simulink model "mech_fceng_vr"  (Simulink 7.1)
settings: Solver=ode45  StartTime=0.0  StopTime=inf  RelTol=1e-3  AbsTol=1e-4
PreLoadFcn:
  | mech_fceng_init;load mech_fceng_images;
InitFcn:
  | mech_slider_open(gcs);
values from neighbouring files (symbols this model uses):
  AirRo = 1.2E-3    (= 0.0012)    [mech_sceng_init.m]
  Cv = 3    [mech_sceng_init.m]
  G = 9.81    [mech_motorcycle_data.m]    (also in mech_sceng_init.m = 1.4)
  Pa = 1033.34    [mech_sceng_init.m]
  Q = 46816    [mech_sceng_init.m]
  R = y([30:p],2)./y([30:p],1)    [mech_car_handling_sweep.m]    (also in mech_flexible_beamelement.m = [1  0  0; mech_sceng_init.m = 5; mech_toroid_setup.m = 10)
  Ta = 25    [mech_sceng_init.m]
  Vo = pi*R*R*14    (= 1099.55742876)    [mech_sceng_init.m]
  Vtdc = pi*R*R*2    (= 157.079632679)    [mech_sceng_init.m]
libraries: mblibv1 x47, simulink x3, simulink_extras x1
(part 2 of 2)

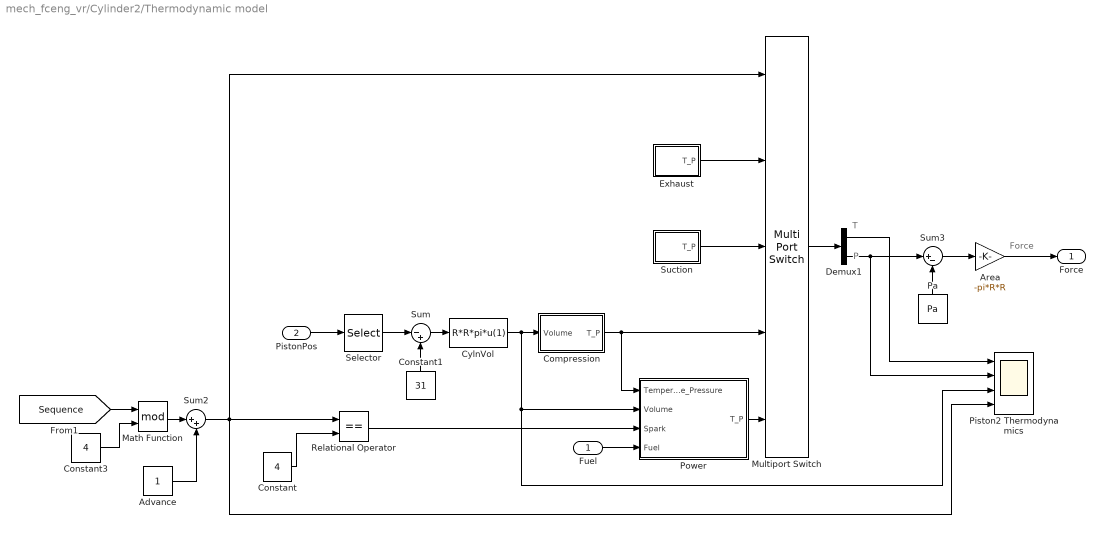
== system mech_fceng_vr/Cylinder2/Thermodynamic model ==
  note: Force
  note: P
  note: T
  Fuel : Inport  OutDataType=sfix(16)  OutScaling=2^0
  PistonPos : Inport  Port=2  OutDataType=sfix(16)  OutScaling=2^0
  Advance : Constant  OutDataType=sfix(16)  OutScaling=2^0
  Area : Gain  Gain=-pi*R*R  ParameterDataType=sfix(16)  ParameterScaling=2^0  OutDataType=sfix(16)  OutScaling=2^0  SaturateOnIntegerOverflow=on  OutDataTypeStr=Inherit: Same as input  ParamDataTypeStr=Inherit: Same as input
  Compression : Subsystem
  Constant : Constant  Value=4  OutDataType=sfix(16)  OutScaling=2^0
  Constant1 : Constant  Orientation=up  Value=31  OutDataType=sfix(16)  OutScaling=2^0
  Constant3 : Constant  Value=4  OutDataType=sfix(16)  OutScaling=2^0
  CylnVol : Fcn  Expr=R*R*pi*u(1)
  Demux1 : Demux  Outputs=2
  Exhaust : Subsystem  TreatAsAtomicUnit=on
  Math Function : Math  Operator=mod  OutDataType=sfix(16)  OutScaling=2^0  SaturateOnIntegerOverflow=on
  Multiport Switch : MultiPortSwitch  Inputs=4  InputSameDT=on
  Pa : Constant  Orientation=up  Value=Pa  OutDataType=sfix(16)  OutScaling=2^0
  Piston2 Thermodynamics : Scope  NumInputPorts=4
      settings: YMin=20~0~0~1  YMax=160~90000~1100~4
  Power : Subsystem
  Relational Operator : RelationalOperator  Operator===  ZeroCross=off  InputSameDT=on
  Selector : Selector  InputPortWidth=3  IndexOptions=Index vector (dialog)  Indices=2  OutputSizes=1
  Suction : Subsystem  TreatAsAtomicUnit=on
  Sum : Sum  Inputs=|-+  OutDataType=sfix(16)  OutScaling=2^0  SaturateOnIntegerOverflow=on  InputSameDT=on  OutDataTypeStr=Inherit: Same as first input
  Sum2 : Sum  Inputs=|++  OutDataType=sfix(16)  OutScaling=2^0  SaturateOnIntegerOverflow=on  InputSameDT=on  OutDataTypeStr=Inherit: Same as first input
  Sum3 : Sum  Inputs=|+-  OutDataType=sfix(16)  OutScaling=2^0  SaturateOnIntegerOverflow=on  InputSameDT=on  OutDataTypeStr=Inherit: Same as first input
  Force : Outport  OutDataType=sfix(16)  OutScaling=2^0
  wires:
  Sum2/1 -> Piston2 Thermodynamics/4, Multiport Switch/1, Relational Operator/1
  [Sequence] -> Math Function/1
  Advance/1 -> Sum2/2
  Math Function/1 -> Sum2/1
  Constant3/1 -> Math Function/2
  PistonPos/1 -> Selector/1
  Selector/1 -> Sum/1
  Relational Operator/1 -> Power/3(Spark)
  Area/1 -> Force/1
  Sum/1 -> CylnVol/1
  Constant/1 -> Relational Operator/2
  Demux1/1 -> Piston2 Thermodynamics/1
  Compression/1(T_P) -> Multiport Switch/4, Power/1(Temperature_Pressure)
  CylnVol/1 -> Piston2 Thermodynamics/3, Power/2(Volume), Compression/1(Volume)
  Constant1/1 -> Sum/2
  Fuel/1 -> Power/4(Fuel)
  Power/1(T_P) -> Multiport Switch/5
  Demux1/2 -> Piston2 Thermodynamics/2, Sum3/1
  Sum3/1 -> Area/1
  Pa/1 -> Sum3/2
  Multiport Switch/1 -> Demux1/1
  Exhaust/1(T_P) -> Multiport Switch/2
  Suction/1(T_P) -> Multiport Switch/3

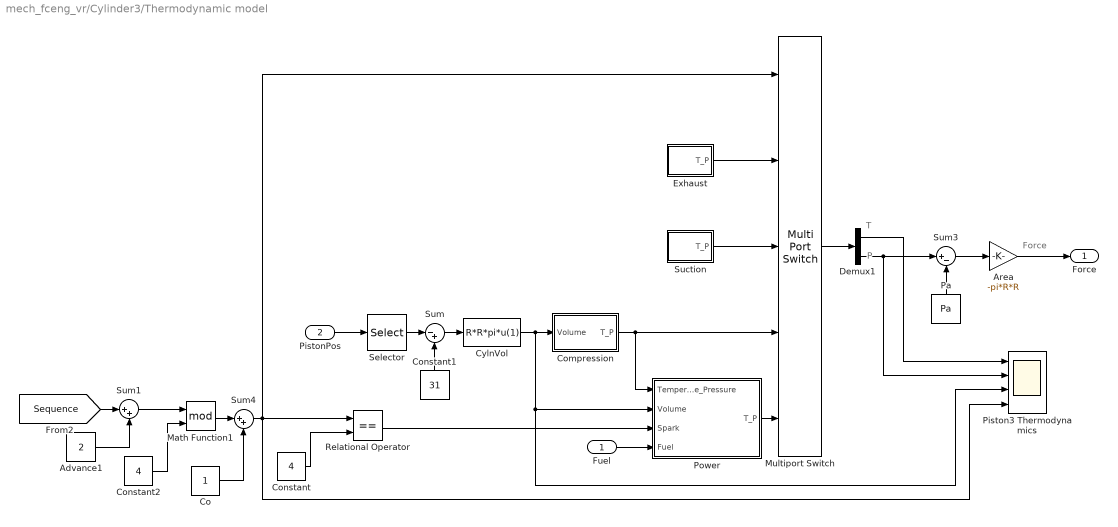
== system mech_fceng_vr/Cylinder3/Thermodynamic model ==
  note: Force
  note: P
  note: T
  Fuel : Inport  OutDataType=sfix(16)  OutScaling=2^0
  PistonPos : Inport  Port=2  OutDataType=sfix(16)  OutScaling=2^0
  Advance1 : Constant  Value=2  OutDataType=sfix(16)  OutScaling=2^0
  Area : Gain  Gain=-pi*R*R  ParameterDataType=sfix(16)  ParameterScaling=2^0  OutDataType=sfix(16)  OutScaling=2^0  SaturateOnIntegerOverflow=on  OutDataTypeStr=Inherit: Same as input  ParamDataTypeStr=Inherit: Same as input
  Co : Constant  OutDataType=sfix(16)  OutScaling=2^0
  Compression : Subsystem
  Constant : Constant  Value=4  OutDataType=sfix(16)  OutScaling=2^0
  Constant1 : Constant  Orientation=up  Value=31  OutDataType=sfix(16)  OutScaling=2^0
  Constant2 : Constant  Value=4  OutDataType=sfix(16)  OutScaling=2^0
  CylnVol : Fcn  Expr=R*R*pi*u(1)
  Demux1 : Demux  Outputs=2
  Exhaust : Subsystem  TreatAsAtomicUnit=on
  Math Function1 : Math  Operator=mod  OutDataType=sfix(16)  OutScaling=2^0  SaturateOnIntegerOverflow=on
  Multiport Switch : MultiPortSwitch  Inputs=4  InputSameDT=on
  Pa : Constant  Orientation=up  Value=Pa  OutDataType=sfix(16)  OutScaling=2^0
  Piston3 Thermodynamics : Scope  NumInputPorts=4
      settings: TimeRange=20  YMin=25~0~0~1  YMax=350~200000~1100~4
  Power : Subsystem
  Relational Operator : RelationalOperator  Operator===  ZeroCross=off  InputSameDT=on
  Selector : Selector  InputPortWidth=3  IndexOptions=Index vector (dialog)  Indices=2  OutputSizes=1
  Suction : Subsystem  TreatAsAtomicUnit=on
  Sum : Sum  Inputs=|-+  OutDataType=sfix(16)  OutScaling=2^0  SaturateOnIntegerOverflow=on  InputSameDT=on  OutDataTypeStr=Inherit: Same as first input
  Sum1 : Sum  Inputs=|++  OutDataType=sfix(16)  OutScaling=2^0  SaturateOnIntegerOverflow=on  InputSameDT=on  OutDataTypeStr=Inherit: Same as first input
  Sum3 : Sum  Inputs=|+-  OutDataType=sfix(16)  OutScaling=2^0  SaturateOnIntegerOverflow=on  InputSameDT=on  OutDataTypeStr=Inherit: Same as first input
  Sum4 : Sum  Inputs=|++  OutDataType=sfix(16)  OutScaling=2^0  SaturateOnIntegerOverflow=on  InputSameDT=on  OutDataTypeStr=Inherit: Same as first input
  Force : Outport  OutDataType=sfix(16)  OutScaling=2^0
  wires:
  Advance1/1 -> Sum1/2
  [Sequence] -> Sum1/1
  Sum1/1 -> Math Function1/1
  Co/1 -> Sum4/2
  Math Function1/1 -> Sum4/1
  Constant2/1 -> Math Function1/2
  Sum4/1 -> Piston3 Thermodynamics/4, Multiport Switch/1, Relational Operator/1
  PistonPos/1 -> Selector/1
  Selector/1 -> Sum/1
  Relational Operator/1 -> Power/3(Spark)
  Area/1 -> Force/1
  Sum/1 -> CylnVol/1
  Constant/1 -> Relational Operator/2
  Demux1/1 -> Piston3 Thermodynamics/1
  Compression/1(T_P) -> Multiport Switch/4, Power/1(Temperature_Pressure)
  CylnVol/1 -> Piston3 Thermodynamics/3, Power/2(Volume), Compression/1(Volume)
  Constant1/1 -> Sum/2
  Fuel/1 -> Power/4(Fuel)
  Power/1(T_P) -> Multiport Switch/5
  Demux1/2 -> Piston3 Thermodynamics/2, Sum3/1
  Sum3/1 -> Area/1
  Pa/1 -> Sum3/2
  Multiport Switch/1 -> Demux1/1
  Exhaust/1(T_P) -> Multiport Switch/2
  Suction/1(T_P) -> Multiport Switch/3

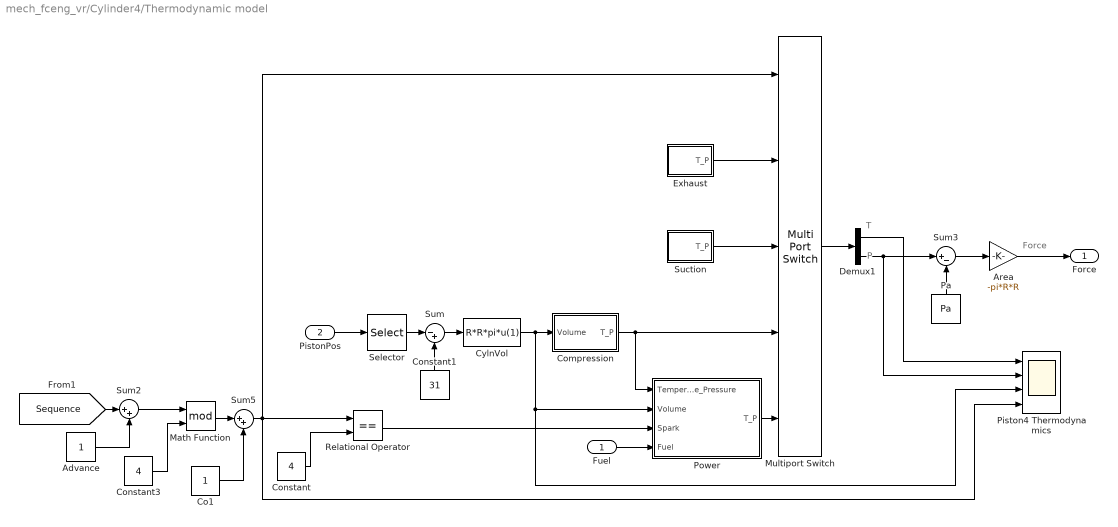
== system mech_fceng_vr/Cylinder4/Thermodynamic model ==
  note: T
  note: P
  note: Force
  Fuel : Inport  OutDataType=sfix(16)  OutScaling=2^0
  PistonPos : Inport  Port=2  OutDataType=sfix(16)  OutScaling=2^0
  Advance : Constant  OutDataType=sfix(16)  OutScaling=2^0
  Area : Gain  Gain=-pi*R*R  ParameterDataType=sfix(16)  ParameterScaling=2^0  OutDataType=sfix(16)  OutScaling=2^0  SaturateOnIntegerOverflow=on  OutDataTypeStr=Inherit: Same as input  ParamDataTypeStr=Inherit: Same as input
  Co1 : Constant  OutDataType=sfix(16)  OutScaling=2^0
  Compression : Subsystem
  Constant : Constant  Value=4  OutDataType=sfix(16)  OutScaling=2^0
  Constant1 : Constant  Orientation=up  Value=31  OutDataType=sfix(16)  OutScaling=2^0
  Constant3 : Constant  Value=4  OutDataType=sfix(16)  OutScaling=2^0
  CylnVol : Fcn  Expr=R*R*pi*u(1)
  Demux1 : Demux  Outputs=2
  Exhaust : Subsystem  TreatAsAtomicUnit=on
  Math Function : Math  Operator=mod  OutDataType=sfix(16)  OutScaling=2^0  SaturateOnIntegerOverflow=on
  Multiport Switch : MultiPortSwitch  Inputs=4  InputSameDT=on
  Pa : Constant  Orientation=up  Value=Pa  OutDataType=sfix(16)  OutScaling=2^0
  Piston4 Thermodynamics : Scope  NumInputPorts=4
      settings: YMin=0~0~0~1  YMax=4500~2.5e+006~1100~4
  Power : Subsystem
  Relational Operator : RelationalOperator  Operator===  ZeroCross=off  InputSameDT=on
  Selector : Selector  InputPortWidth=3  IndexOptions=Index vector (dialog)  Indices=2  OutputSizes=1
  Suction : Subsystem  TreatAsAtomicUnit=on
  Sum : Sum  Inputs=|-+  OutDataType=sfix(16)  OutScaling=2^0  SaturateOnIntegerOverflow=on  InputSameDT=on  OutDataTypeStr=Inherit: Same as first input
  Sum2 : Sum  Inputs=|++  OutDataType=sfix(16)  OutScaling=2^0  SaturateOnIntegerOverflow=on  InputSameDT=on  OutDataTypeStr=Inherit: Same as first input
  Sum3 : Sum  Inputs=|+-  OutDataType=sfix(16)  OutScaling=2^0  SaturateOnIntegerOverflow=on  InputSameDT=on  OutDataTypeStr=Inherit: Same as first input
  Sum5 : Sum  Inputs=|++  OutDataType=sfix(16)  OutScaling=2^0  SaturateOnIntegerOverflow=on  InputSameDT=on  OutDataTypeStr=Inherit: Same as first input
  Force : Outport  OutDataType=sfix(16)  OutScaling=2^0
  wires:
  Advance/1 -> Sum2/2
  [Sequence] -> Sum2/1
  Sum2/1 -> Math Function/1
  Co1/1 -> Sum5/2
  Math Function/1 -> Sum5/1
  Constant3/1 -> Math Function/2
  Suction/1(T_P) -> Multiport Switch/3
  Exhaust/1(T_P) -> Multiport Switch/2
  Multiport Switch/1 -> Demux1/1
  Pa/1 -> Sum3/2
  Sum3/1 -> Area/1
  Demux1/2 -> Sum3/1, Piston4 Thermodynamics/2
  Power/1(T_P) -> Multiport Switch/5
  Fuel/1 -> Power/4(Fuel)
  Constant1/1 -> Sum/2
  CylnVol/1 -> Compression/1(Volume), Power/2(Volume), Piston4 Thermodynamics/3
  Compression/1(T_P) -> Power/1(Temperature_Pressure), Multiport Switch/4
  Demux1/1 -> Piston4 Thermodynamics/1
  Constant/1 -> Relational Operator/2
  Sum/1 -> CylnVol/1
  Area/1 -> Force/1
  Relational Operator/1 -> Power/3(Spark)
  Selector/1 -> Sum/1
  PistonPos/1 -> Selector/1
  Sum5/1 -> Piston4 Thermodynamics/4, Relational Operator/1, Multiport Switch/1

== system mech_fceng_vr/Engine Block/Engine Timer ==
  Angle : Inport  Orientation=left  OutDataType=sfix(16)  OutScaling=2^0
  Constant : Constant  Orientation=left  Value=pi/4  OutDataType=sfix(16)  OutScaling=2^0
  Hit  Crossing2 : HitCross  Orientation=left  ZeroCross=off
  Ignition Control : Stateflow chart  Orientation=left  TreatAsAtomicUnit=on
  Sum : Sum  Orientation=left  Inputs=++|  OutDataType=sfix(16)  OutScaling=2^0  SaturateOnIntegerOverflow=on  InputSameDT=on  OutDataTypeStr=Inherit: Same as first input
  Trigonometric Function : Trigonometry  Orientation=left  Operator=cos
  tag scope: Sequence=global
  wires:
  Ignition Control/1(Sequence) -> [Sequence]
  Hit  Crossing2/1 -> Ignition Control/Trigger
  Trigonometric Function/1 -> Hit  Crossing2/1
  Sum/1 -> Ignition Control/1(CrankAngle), Trigonometric Function/1
  Constant/1 -> Sum/1
  Angle/1 -> Sum/2

== system mech_fceng_vr/Engine Block/Friction ==
  Angle : Inport  Orientation=left  OutDataType=sfix(16)  OutScaling=2^0
  Rate : Inport  Orientation=left  Port=2  OutDataType=sfix(16)  OutScaling=2^0
  Fcn : Fcn  Orientation=left  Expr=u < 0
  Gain : Gain  Orientation=left  Gain=1000  ParameterDataType=sfix(16)  ParameterScaling=2^0  OutDataType=sfix(16)  OutScaling=2^0  SaturateOnIntegerOverflow=on  OutDataTypeStr=Inherit: Same as input  ParamDataTypeStr=Inherit: Same as input
  Gain1 : Gain  Orientation=left  Gain=-200  ParameterDataType=sfix(16)  ParameterScaling=2^0  OutDataType=sfix(16)  OutScaling=2^0  SaturateOnIntegerOverflow=on  OutDataTypeStr=Inherit: Same as input  ParamDataTypeStr=Inherit: Same as input
  S-R Flip-Flop : simulink_extras/Flip Flops/S-R Flip-Flop  Orientation=left  SystemSampleTime=-1  initial_condition=0
  Sum1 : Sum  Orientation=left  Inputs=++|  OutDataType=sfix(16)  OutScaling=2^0  SaturateOnIntegerOverflow=on  InputSameDT=on  OutDataTypeStr=Inherit: Same as first input
  Torque : Outport  Orientation=left  OutDataType=sfix(16)  OutScaling=2^0
  tag scope: CrankSR=global
  wires:
  Sum1/1 -> Torque/1
  Angle/1 -> [CrankSR], Fcn/1
  Rate/1 -> Gain1/1
  Gain1/1 -> Sum1/1
  Gain/1 -> Sum1/2
  S-R Flip-Flop/2 -> Gain/1
  Fcn/1 -> S-R Flip-Flop/1

== system mech_fceng_vr/Cylinder1/Thermodynamic model/Compression ==
  note: Compression
  note: P
  note: T
  Volume : Inport  OutDataType=sfix(16)  OutScaling=2^0
  Mux : Mux  Inputs=2
  P : Fcn  Expr=Pa*(Vo/u(1))^G
  T : Fcn  Expr=Ta*(Vo/u(1))^(G-1)
  T_P : Outport  OutDataType=sfix(16)  OutScaling=2^0
  wires:
  Volume/1 -> P/1, T/1
  Mux/1 -> T_P/1
  P/1 -> Mux/2
  T/1 -> Mux/1

== system mech_fceng_vr/Cylinder1/Thermodynamic model/Exhaust ==
  note: Exhaust
  Mux : Mux  Inputs=2
  Pa : Constant  Value=Pa  OutDataType=sfix(16)  OutScaling=2^0
  Ta : Constant  Value=Ta  OutDataType=sfix(16)  OutScaling=2^0
  T_P : Outport  OutDataType=sfix(16)  OutScaling=2^0
  wires:
  Mux/1 -> T_P/1
  Ta/1 -> Mux/1
  Pa/1 -> Mux/2

== system mech_fceng_vr/Cylinder1/Thermodynamic model/Power ==
  Temperature_Pressure : Inport  OutDataType=sfix(16)  OutScaling=2^0
  Volume : Inport  Port=2  OutDataType=sfix(16)  OutScaling=2^0
  Spark : Inport  Port=3  OutDataType=sfix(16)  OutScaling=2^0
  Fuel : Inport  Port=4  OutDataType=sfix(16)  OutScaling=2^0
  Combustion : Subsystem  TreatAsAtomicUnit=on
  Demux1 : Demux  Outputs=2
  IC : InitialCondition  Value=[Ta;Pa]
  IdealExpansion : Subsystem  TreatAsAtomicUnit=on
  Mux : Mux  Inputs=2
  T_P : Outport  OutDataType=sfix(16)  OutScaling=2^0
  wires:
  Combustion/3(VolumeAfterCombustion) -> IdealExpansion/3(VolumeAfterCombustion)
  Combustion/1(TemperatureAfterCombustion) -> IdealExpansion/1(TemperatureAfterCombustion)
  IC/1 -> Demux1/1
  IdealExpansion/2(FPressure) -> Mux/2
  IdealExpansion/1(FTemperature) -> Mux/1
  Volume/1 -> Combustion/4(VolumeBeforeCombustion), IdealExpansion/4(IVolume)
  Combustion/2(PressureAfterCombustion) -> IdealExpansion/2(PressureAfterCombustion)
  Demux1/2 -> Combustion/2(PressureBeforeCombustion)
  Demux1/1 -> Combustion/1(TemperatureBeforeCombustion)
  Temperature_Pressure/1 -> IC/1
  Spark/1 -> Combustion/Trigger
  Fuel/1 -> Combustion/3(Fuel)
  Mux/1 -> T_P/1

== system mech_fceng_vr/Cylinder1/Thermodynamic model/Suction ==
  note: Suction
  Mux : Mux  Inputs=2
  Pa : Constant  Value=Pa  OutDataType=sfix(16)  OutScaling=2^0
  Ta : Constant  Value=Ta  OutDataType=sfix(16)  OutScaling=2^0
  T_P : Outport  OutDataType=sfix(16)  OutScaling=2^0
  wires:
  Pa/1 -> Mux/2
  Ta/1 -> Mux/1
  Mux/1 -> T_P/1

== system mech_fceng_vr/Cylinder2/Thermodynamic model/Compression ==
  note: Compression
  note: P
  note: T
  Volume : Inport  OutDataType=sfix(16)  OutScaling=2^0
  Mux : Mux  Inputs=2
  P : Fcn  Expr=Pa*(Vo/u(1))^G
  T : Fcn  Expr=Ta*(Vo/u(1))^(G-1)
  T_P : Outport  OutDataType=sfix(16)  OutScaling=2^0
  wires:
  Volume/1 -> P/1, T/1
  Mux/1 -> T_P/1
  P/1 -> Mux/2
  T/1 -> Mux/1

== system mech_fceng_vr/Cylinder2/Thermodynamic model/Exhaust ==
  note: Exhaust
  Mux : Mux  Inputs=2
  Pa : Constant  Value=Pa  OutDataType=sfix(16)  OutScaling=2^0
  Ta : Constant  Value=Ta  OutDataType=sfix(16)  OutScaling=2^0
  T_P : Outport  OutDataType=sfix(16)  OutScaling=2^0
  wires:
  Mux/1 -> T_P/1
  Ta/1 -> Mux/1
  Pa/1 -> Mux/2

== system mech_fceng_vr/Cylinder2/Thermodynamic model/Power ==
  Temperature_Pressure : Inport  OutDataType=sfix(16)  OutScaling=2^0
  Volume : Inport  Port=2  OutDataType=sfix(16)  OutScaling=2^0
  Spark : Inport  Port=3  OutDataType=sfix(16)  OutScaling=2^0
  Fuel : Inport  Port=4  OutDataType=sfix(16)  OutScaling=2^0
  Combustion : Subsystem  TreatAsAtomicUnit=on
  Demux1 : Demux  Outputs=2
  IC : InitialCondition  Value=[Ta;Pa]
  IdealExpansion : Subsystem  TreatAsAtomicUnit=on
  Mux : Mux  Inputs=2
  T_P : Outport  OutDataType=sfix(16)  OutScaling=2^0
  wires:
  IC/1 -> Demux1/1
  IdealExpansion/2(FPressure) -> Mux/2
  IdealExpansion/1(FTemperature) -> Mux/1
  Volume/1 -> Combustion/4(VolumeBeforeCombustion), IdealExpansion/4(IVolume)
  Combustion/3(VolumeAfterCombustion) -> IdealExpansion/3(VolumeAfterCombustion)
  Combustion/2(PressureAfterCombustion) -> IdealExpansion/2(PressureAfterCombustion)
  Combustion/1(TemperatureAfterCombustion) -> IdealExpansion/1(TemperatureAfterCombustion)
  Demux1/2 -> Combustion/2(PressureBeforeCombustion)
  Demux1/1 -> Combustion/1(TemperatureBeforeCombustion)
  Temperature_Pressure/1 -> IC/1
  Spark/1 -> Combustion/Trigger
  Fuel/1 -> Combustion/3(Fuel)
  Mux/1 -> T_P/1

== system mech_fceng_vr/Cylinder2/Thermodynamic model/Suction ==
  note: Suction
  Mux : Mux  Inputs=2
  Pa : Constant  Value=Pa  OutDataType=sfix(16)  OutScaling=2^0
  Ta : Constant  Value=Ta  OutDataType=sfix(16)  OutScaling=2^0
  T_P : Outport  OutDataType=sfix(16)  OutScaling=2^0
  wires:
  Pa/1 -> Mux/2
  Ta/1 -> Mux/1
  Mux/1 -> T_P/1

== system mech_fceng_vr/Cylinder3/Thermodynamic model/Compression ==
  note: Compression
  note: P
  note: T
  Volume : Inport  OutDataType=sfix(16)  OutScaling=2^0
  Mux : Mux  Inputs=2
  P : Fcn  Expr=Pa*(Vo/u(1))^G
  T : Fcn  Expr=Ta*(Vo/u(1))^(G-1)
  T_P : Outport  OutDataType=sfix(16)  OutScaling=2^0
  wires:
  Volume/1 -> P/1, T/1
  Mux/1 -> T_P/1
  P/1 -> Mux/2
  T/1 -> Mux/1

== system mech_fceng_vr/Cylinder3/Thermodynamic model/Exhaust ==
  note: Exhaust
  Mux : Mux  Inputs=2
  Pa : Constant  Value=Pa  OutDataType=sfix(16)  OutScaling=2^0
  Ta : Constant  Value=Ta  OutDataType=sfix(16)  OutScaling=2^0
  T_P : Outport  OutDataType=sfix(16)  OutScaling=2^0
  wires:
  Mux/1 -> T_P/1
  Ta/1 -> Mux/1
  Pa/1 -> Mux/2

== system mech_fceng_vr/Cylinder3/Thermodynamic model/Power ==
  Temperature_Pressure : Inport  OutDataType=sfix(16)  OutScaling=2^0
  Volume : Inport  Port=2  OutDataType=sfix(16)  OutScaling=2^0
  Spark : Inport  Port=3  OutDataType=sfix(16)  OutScaling=2^0
  Fuel : Inport  Port=4  OutDataType=sfix(16)  OutScaling=2^0
  Combustion : Subsystem  TreatAsAtomicUnit=on
  Demux1 : Demux  Outputs=2
  IC : InitialCondition  Value=[Ta;Pa]
  IdealExpansion : Subsystem  TreatAsAtomicUnit=on
  Mux : Mux  Inputs=2
  T_P : Outport  OutDataType=sfix(16)  OutScaling=2^0
  wires:
  IC/1 -> Demux1/1
  IdealExpansion/2(FPressure) -> Mux/2
  IdealExpansion/1(FTemperature) -> Mux/1
  Volume/1 -> Combustion/4(VolumeBeforeCombustion), IdealExpansion/4(IVolume)
  Combustion/3(VolumeAfterCombustion) -> IdealExpansion/3(VolumeAfterCombustion)
  Combustion/2(PressureAfterCombustion) -> IdealExpansion/2(PressureAfterCombustion)
  Combustion/1(TemperatureAfterCombustion) -> IdealExpansion/1(TemperatureAfterCombustion)
  Demux1/2 -> Combustion/2(PressureBeforeCombustion)
  Demux1/1 -> Combustion/1(TemperatureBeforeCombustion)
  Temperature_Pressure/1 -> IC/1
  Spark/1 -> Combustion/Trigger
  Fuel/1 -> Combustion/3(Fuel)
  Mux/1 -> T_P/1

== system mech_fceng_vr/Cylinder3/Thermodynamic model/Suction ==
  note: Suction
  Mux : Mux  Inputs=2
  Pa : Constant  Value=Pa  OutDataType=sfix(16)  OutScaling=2^0
  Ta : Constant  Value=Ta  OutDataType=sfix(16)  OutScaling=2^0
  T_P : Outport  OutDataType=sfix(16)  OutScaling=2^0
  wires:
  Pa/1 -> Mux/2
  Ta/1 -> Mux/1
  Mux/1 -> T_P/1

== system mech_fceng_vr/Cylinder4/Thermodynamic model/Compression ==
  note: T
  note: P
  note: Compression
  Volume : Inport  OutDataType=sfix(16)  OutScaling=2^0
  Mux : Mux  Inputs=2
  P : Fcn  Expr=Pa*(Vo/u(1))^G
  T : Fcn  Expr=Ta*(Vo/u(1))^(G-1)
  T_P : Outport  OutDataType=sfix(16)  OutScaling=2^0
  wires:
  T/1 -> Mux/1
  P/1 -> Mux/2
  Mux/1 -> T_P/1
  Volume/1 -> T/1, P/1

== system mech_fceng_vr/Cylinder4/Thermodynamic model/Exhaust ==
  note: Exhaust
  Mux : Mux  Inputs=2
  Pa : Constant  Value=Pa  OutDataType=sfix(16)  OutScaling=2^0
  Ta : Constant  Value=Ta  OutDataType=sfix(16)  OutScaling=2^0
  T_P : Outport  OutDataType=sfix(16)  OutScaling=2^0
  wires:
  Pa/1 -> Mux/2
  Ta/1 -> Mux/1
  Mux/1 -> T_P/1

== system mech_fceng_vr/Cylinder4/Thermodynamic model/Power ==
  Temperature_Pressure : Inport  OutDataType=sfix(16)  OutScaling=2^0
  Volume : Inport  Port=2  OutDataType=sfix(16)  OutScaling=2^0
  Spark : Inport  Port=3  OutDataType=sfix(16)  OutScaling=2^0
  Fuel : Inport  Port=4  OutDataType=sfix(16)  OutScaling=2^0
  Combustion : Subsystem  TreatAsAtomicUnit=on
  Demux1 : Demux  Outputs=2
  IC : InitialCondition  Value=[Ta;Pa]
  IdealExpansion : Subsystem  TreatAsAtomicUnit=on
  Mux : Mux  Inputs=2
  T_P : Outport  OutDataType=sfix(16)  OutScaling=2^0
  wires:
  Mux/1 -> T_P/1
  Fuel/1 -> Combustion/3(Fuel)
  Spark/1 -> Combustion/Trigger
  Temperature_Pressure/1 -> IC/1
  Demux1/1 -> Combustion/1(TemperatureBeforeCombustion)
  Demux1/2 -> Combustion/2(PressureBeforeCombustion)
  Combustion/1(TemperatureAfterCombustion) -> IdealExpansion/1(TemperatureAfterCombustion)
  Combustion/2(PressureAfterCombustion) -> IdealExpansion/2(PressureAfterCombustion)
  Combustion/3(VolumeAfterCombustion) -> IdealExpansion/3(VolumeAfterCombustion)
  Volume/1 -> IdealExpansion/4(IVolume), Combustion/4(VolumeBeforeCombustion)
  IdealExpansion/1(FTemperature) -> Mux/1
  IdealExpansion/2(FPressure) -> Mux/2
  IC/1 -> Demux1/1

== system mech_fceng_vr/Cylinder4/Thermodynamic model/Suction ==
  note: Suction
  Mux : Mux  Inputs=2
  Pa : Constant  Value=Pa  OutDataType=sfix(16)  OutScaling=2^0
  Ta : Constant  Value=Ta  OutDataType=sfix(16)  OutScaling=2^0
  T_P : Outport  OutDataType=sfix(16)  OutScaling=2^0
  wires:
  Mux/1 -> T_P/1
  Ta/1 -> Mux/1
  Pa/1 -> Mux/2

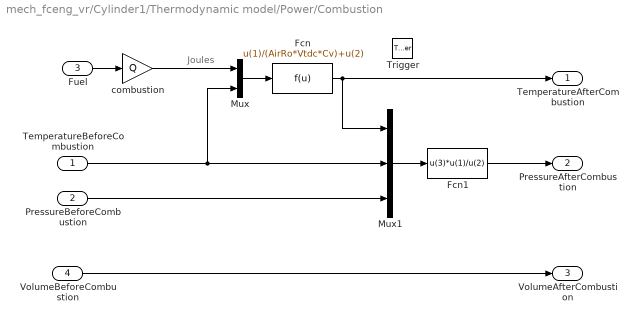
== system mech_fceng_vr/Cylinder1/Thermodynamic model/Power/Combustion ==
  note: Joules
  TemperatureBeforeCombustion : Inport  OutDataType=sfix(16)  OutScaling=2^0
  PressureBeforeCombustion : Inport  Port=2  OutDataType=sfix(16)  OutScaling=2^0
  Fuel : Inport  Port=3  OutDataType=sfix(16)  OutScaling=2^0
  VolumeBeforeCombustion : Inport  Port=4  OutDataType=sfix(16)  OutScaling=2^0
  Trigger : TriggerPort  ZeroCross=off
  Fcn : Fcn  Expr=u(1)/(AirRo*Vtdc*Cv)+u(2)
  Fcn1 : Fcn  Expr=u(3)*u(1)/u(2)
  Mux : Mux  Inputs=2
  Mux1 : Mux  Inputs=3
  combustion : Gain  Gain=Q  ParameterDataType=sfix(16)  ParameterScaling=2^0  OutDataType=sfix(16)  OutScaling=2^0  SaturateOnIntegerOverflow=on  OutDataTypeStr=Inherit: Same as input  ParamDataTypeStr=Inherit: Same as input
  TemperatureAfterCombustion : Outport  OutDataType=sfix(16)  OutScaling=2^0
  PressureAfterCombustion : Outport  Port=2  OutDataType=sfix(16)  OutScaling=2^0
  VolumeAfterCombustion : Outport  Port=3  OutDataType=sfix(16)  OutScaling=2^0
  wires:
  VolumeBeforeCombustion/1 -> VolumeAfterCombustion/1
  Fuel/1 -> combustion/1
  combustion/1 -> Mux/1
  TemperatureBeforeCombustion/1 -> Mux1/2, Mux/2
  Mux1/1 -> Fcn1/1
  PressureBeforeCombustion/1 -> Mux1/3
  Fcn1/1 -> PressureAfterCombustion/1
  Fcn/1 -> TemperatureAfterCombustion/1, Mux1/1
  Mux/1 -> Fcn/1

== system mech_fceng_vr/Cylinder1/Thermodynamic model/Power/IdealExpansion ==
  TemperatureAfterCombustion : Inport  OutDataType=sfix(16)  OutScaling=2^0
  PressureAfterCombustion : Inport  Port=2  OutDataType=sfix(16)  OutScaling=2^0
  VolumeAfterCombustion : Inport  Port=3  OutDataType=sfix(16)  OutScaling=2^0
  IVolume : Inport  Port=4  OutDataType=sfix(16)  OutScaling=2^0
  Mux : Mux  Inputs=3
  Mux1 : Mux  Inputs=3
  P : Fcn  Expr=u(1)*(u(3)/u(2))^G
  T : Fcn  Expr=u(1)*(u(3)/u(2))^(G-1)
  FTemperature : Outport  OutDataType=sfix(16)  OutScaling=2^0
  FPressure : Outport  Port=2  OutDataType=sfix(16)  OutScaling=2^0
  wires:
  VolumeAfterCombustion/1 -> Mux/3, Mux1/3
  IVolume/1 -> Mux/2, Mux1/2
  PressureAfterCombustion/1 -> Mux1/1
  P/1 -> FPressure/1
  Mux1/1 -> P/1
  T/1 -> FTemperature/1
  Mux/1 -> T/1
  TemperatureAfterCombustion/1 -> Mux/1

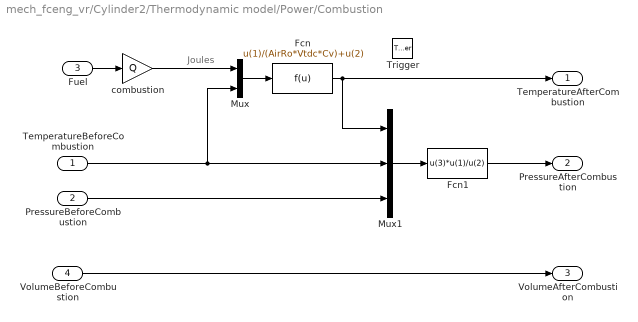
== system mech_fceng_vr/Cylinder2/Thermodynamic model/Power/Combustion ==
  note: Joules
  TemperatureBeforeCombustion : Inport  OutDataType=sfix(16)  OutScaling=2^0
  PressureBeforeCombustion : Inport  Port=2  OutDataType=sfix(16)  OutScaling=2^0
  Fuel : Inport  Port=3  OutDataType=sfix(16)  OutScaling=2^0
  VolumeBeforeCombustion : Inport  Port=4  OutDataType=sfix(16)  OutScaling=2^0
  Trigger : TriggerPort  ZeroCross=off
  Fcn : Fcn  Expr=u(1)/(AirRo*Vtdc*Cv)+u(2)
  Fcn1 : Fcn  Expr=u(3)*u(1)/u(2)
  Mux : Mux  Inputs=2
  Mux1 : Mux  Inputs=3
  combustion : Gain  Gain=Q  ParameterDataType=sfix(16)  ParameterScaling=2^0  OutDataType=sfix(16)  OutScaling=2^0  SaturateOnIntegerOverflow=on  OutDataTypeStr=Inherit: Same as input  ParamDataTypeStr=Inherit: Same as input
  TemperatureAfterCombustion : Outport  OutDataType=sfix(16)  OutScaling=2^0
  PressureAfterCombustion : Outport  Port=2  OutDataType=sfix(16)  OutScaling=2^0
  VolumeAfterCombustion : Outport  Port=3  OutDataType=sfix(16)  OutScaling=2^0
  wires:
  VolumeBeforeCombustion/1 -> VolumeAfterCombustion/1
  Fuel/1 -> combustion/1
  combustion/1 -> Mux/1
  TemperatureBeforeCombustion/1 -> Mux1/2, Mux/2
  Mux1/1 -> Fcn1/1
  PressureBeforeCombustion/1 -> Mux1/3
  Fcn1/1 -> PressureAfterCombustion/1
  Fcn/1 -> TemperatureAfterCombustion/1, Mux1/1
  Mux/1 -> Fcn/1

== system mech_fceng_vr/Cylinder2/Thermodynamic model/Power/IdealExpansion ==
  TemperatureAfterCombustion : Inport  OutDataType=sfix(16)  OutScaling=2^0
  PressureAfterCombustion : Inport  Port=2  OutDataType=sfix(16)  OutScaling=2^0
  VolumeAfterCombustion : Inport  Port=3  OutDataType=sfix(16)  OutScaling=2^0
  IVolume : Inport  Port=4  OutDataType=sfix(16)  OutScaling=2^0
  Mux : Mux  Inputs=3
  Mux1 : Mux  Inputs=3
  P : Fcn  Expr=u(1)*(u(3)/u(2))^G
  T : Fcn  Expr=u(1)*(u(3)/u(2))^(G-1)
  FTemperature : Outport  OutDataType=sfix(16)  OutScaling=2^0
  FPressure : Outport  Port=2  OutDataType=sfix(16)  OutScaling=2^0
  wires:
  VolumeAfterCombustion/1 -> Mux/3, Mux1/3
  IVolume/1 -> Mux/2, Mux1/2
  PressureAfterCombustion/1 -> Mux1/1
  P/1 -> FPressure/1
  Mux1/1 -> P/1
  T/1 -> FTemperature/1
  Mux/1 -> T/1
  TemperatureAfterCombustion/1 -> Mux/1

== system mech_fceng_vr/Cylinder3/Thermodynamic model/Power/Combustion ==
  note: Joules
  TemperatureBeforeCombustion : Inport  OutDataType=sfix(16)  OutScaling=2^0
  PressureBeforeCombustion : Inport  Port=2  OutDataType=sfix(16)  OutScaling=2^0
  Fuel : Inport  Port=3  OutDataType=sfix(16)  OutScaling=2^0
  VolumeBeforeCombustion : Inport  Port=4  OutDataType=sfix(16)  OutScaling=2^0
  Trigger : TriggerPort  ZeroCross=off
  Fcn : Fcn  Expr=u(1)/(AirRo*Vtdc*Cv)+u(2)
  Fcn1 : Fcn  Expr=u(3)*u(1)/u(2)
  Mux : Mux  Inputs=2
  Mux1 : Mux  Inputs=3
  combustion : Gain  Gain=Q  ParameterDataType=sfix(16)  ParameterScaling=2^0  OutDataType=sfix(16)  OutScaling=2^0  SaturateOnIntegerOverflow=on  OutDataTypeStr=Inherit: Same as input  ParamDataTypeStr=Inherit: Same as input
  TemperatureAfterCombustion : Outport  OutDataType=sfix(16)  OutScaling=2^0
  PressureAfterCombustion : Outport  Port=2  OutDataType=sfix(16)  OutScaling=2^0
  VolumeAfterCombustion : Outport  Port=3  OutDataType=sfix(16)  OutScaling=2^0
  wires:
  VolumeBeforeCombustion/1 -> VolumeAfterCombustion/1
  Fuel/1 -> combustion/1
  combustion/1 -> Mux/1
  TemperatureBeforeCombustion/1 -> Mux1/2, Mux/2
  Mux1/1 -> Fcn1/1
  PressureBeforeCombustion/1 -> Mux1/3
  Fcn1/1 -> PressureAfterCombustion/1
  Fcn/1 -> TemperatureAfterCombustion/1, Mux1/1
  Mux/1 -> Fcn/1

== system mech_fceng_vr/Cylinder3/Thermodynamic model/Power/IdealExpansion ==
  TemperatureAfterCombustion : Inport  OutDataType=sfix(16)  OutScaling=2^0
  PressureAfterCombustion : Inport  Port=2  OutDataType=sfix(16)  OutScaling=2^0
  VolumeAfterCombustion : Inport  Port=3  OutDataType=sfix(16)  OutScaling=2^0
  IVolume : Inport  Port=4  OutDataType=sfix(16)  OutScaling=2^0
  Mux : Mux  Inputs=3
  Mux1 : Mux  Inputs=3
  P : Fcn  Expr=u(1)*(u(3)/u(2))^G
  T : Fcn  Expr=u(1)*(u(3)/u(2))^(G-1)
  FTemperature : Outport  OutDataType=sfix(16)  OutScaling=2^0
  FPressure : Outport  Port=2  OutDataType=sfix(16)  OutScaling=2^0
  wires:
  VolumeAfterCombustion/1 -> Mux/3, Mux1/3
  IVolume/1 -> Mux/2, Mux1/2
  PressureAfterCombustion/1 -> Mux1/1
  P/1 -> FPressure/1
  Mux1/1 -> P/1
  T/1 -> FTemperature/1
  Mux/1 -> T/1
  TemperatureAfterCombustion/1 -> Mux/1

== system mech_fceng_vr/Cylinder4/Thermodynamic model/Power/Combustion ==
  note: Joules
  TemperatureBeforeCombustion : Inport  OutDataType=sfix(16)  OutScaling=2^0
  PressureBeforeCombustion : Inport  Port=2  OutDataType=sfix(16)  OutScaling=2^0
  Fuel : Inport  Port=3  OutDataType=sfix(16)  OutScaling=2^0
  VolumeBeforeCombustion : Inport  Port=4  OutDataType=sfix(16)  OutScaling=2^0
  Trigger : TriggerPort  ZeroCross=off
  Fcn : Fcn  Expr=u(1)/(AirRo*Vtdc*Cv)+u(2)
  Fcn1 : Fcn  Expr=u(3)*u(1)/u(2)
  Mux : Mux  Inputs=2
  Mux1 : Mux  Inputs=3
  combustion : Gain  Gain=Q  ParameterDataType=sfix(16)  ParameterScaling=2^0  OutDataType=sfix(16)  OutScaling=2^0  SaturateOnIntegerOverflow=on  OutDataTypeStr=Inherit: Same as input  ParamDataTypeStr=Inherit: Same as input
  TemperatureAfterCombustion : Outport  OutDataType=sfix(16)  OutScaling=2^0
  PressureAfterCombustion : Outport  Port=2  OutDataType=sfix(16)  OutScaling=2^0
  VolumeAfterCombustion : Outport  Port=3  OutDataType=sfix(16)  OutScaling=2^0
  wires:
  Mux/1 -> Fcn/1
  Fcn/1 -> Mux1/1, TemperatureAfterCombustion/1
  Fcn1/1 -> PressureAfterCombustion/1
  PressureBeforeCombustion/1 -> Mux1/3
  Mux1/1 -> Fcn1/1
  TemperatureBeforeCombustion/1 -> Mux/2, Mux1/2
  combustion/1 -> Mux/1
  Fuel/1 -> combustion/1
  VolumeBeforeCombustion/1 -> VolumeAfterCombustion/1

== system mech_fceng_vr/Cylinder4/Thermodynamic model/Power/IdealExpansion ==
  TemperatureAfterCombustion : Inport  OutDataType=sfix(16)  OutScaling=2^0
  PressureAfterCombustion : Inport  Port=2  OutDataType=sfix(16)  OutScaling=2^0
  VolumeAfterCombustion : Inport  Port=3  OutDataType=sfix(16)  OutScaling=2^0
  IVolume : Inport  Port=4  OutDataType=sfix(16)  OutScaling=2^0
  Mux : Mux  Inputs=3
  Mux1 : Mux  Inputs=3
  P : Fcn  Expr=u(1)*(u(3)/u(2))^G
  T : Fcn  Expr=u(1)*(u(3)/u(2))^(G-1)
  FTemperature : Outport  OutDataType=sfix(16)  OutScaling=2^0
  FPressure : Outport  Port=2  OutDataType=sfix(16)  OutScaling=2^0
  wires:
  TemperatureAfterCombustion/1 -> Mux/1
  Mux/1 -> T/1
  T/1 -> FTemperature/1
  Mux1/1 -> P/1
  P/1 -> FPressure/1
  PressureAfterCombustion/1 -> Mux1/1
  IVolume/1 -> Mux1/2, Mux/2
  VolumeAfterCombustion/1 -> Mux1/3, Mux/3

== stateflow chart Engine Block/Engine Timer/Ignition Control ==
  settings: executeAtInitialization=1
  state Ignition_sequence
    state Exhaust
      entry: Sequence = 1;
    state Suction
      entry:Sequence = 2;
    state Compression
      entry:Sequence = 3;
    state Ignition
      entry:Sequence = 4;
    Exhaust -> Suction : [ guard() ]
    Suction -> Compression : [ guard() ]
    Compression -> Ignition : [ guard() ]
    Ignition -> Exhaust : [ guard() ]
  state yes = guard() [function]
    (default) -> (junction 9) : { yes = (abs(CrankAngle - lastCrankAngle) >  0.2);
        |   lastCrankAngle = CrankAngle; }
  (default) -> Exhaust
  data: yes function_output double; lastCrankAngle local double; Sequence output double =1; CrankAngle input double
  events: CrankTrigger input RISING_EDGE_EVENT
